simulink subsystem "F550_Dynamics_sub"  (R2024a)
settings: Solver=VariableStepAuto  StartTime=0.0  StopTime=10.0  RelTol=1e-3
undefined symbols (not defined in the file): armLength, Cd, Cmd, contact, control, ddx, ddy, ddz, dx, dy, dz, dzcg, g, Inertia, Inertia_inv, Mass, motorCr, motorJm, motorRpm0, motorTm, motorWb, p, pitch, q, r, roll, rotorCm, rotorCt, X, x0, Y, yaw, Z
libraries: matrix_library x2, shared6dof x1, simulink x1
settings Model: Creator=CNU_UASG  LastModifiedBy=CNU_UASG

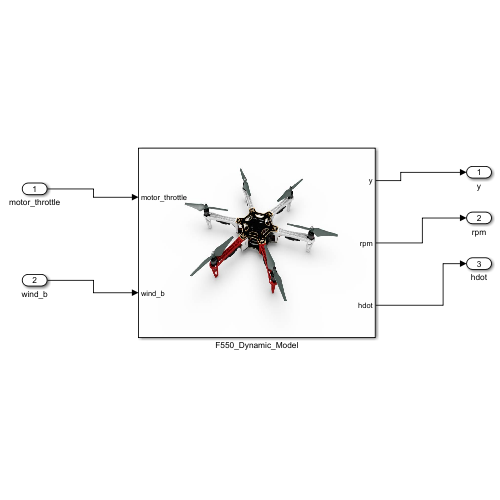
[thumbnail: Simulink's stored preview of the top-level diagram]
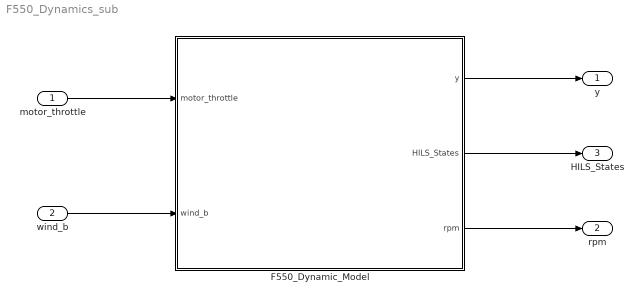
== system F550_Dynamics_sub ==
  motor_throttle : Inport
  wind_b : Inport  Port=2  PortDimensions=[3 1]
  F550_Dynamic_Model : Subsystem
      mask Display: image('F550.jpg');
  y : Outport
  rpm : Outport  Port=2
  HILS_States : Outport  Port=3
  wires:
  F550_Dynamic_Model/1(y) -> y/1
  F550_Dynamic_Model/3(rpm) -> rpm/1
  motor_throttle/1 -> F550_Dynamic_Model/1(motor_throttle)
  wind_b/1 -> F550_Dynamic_Model/2(wind_b)
  F550_Dynamic_Model/2(HILS_States) -> HILS_States/1

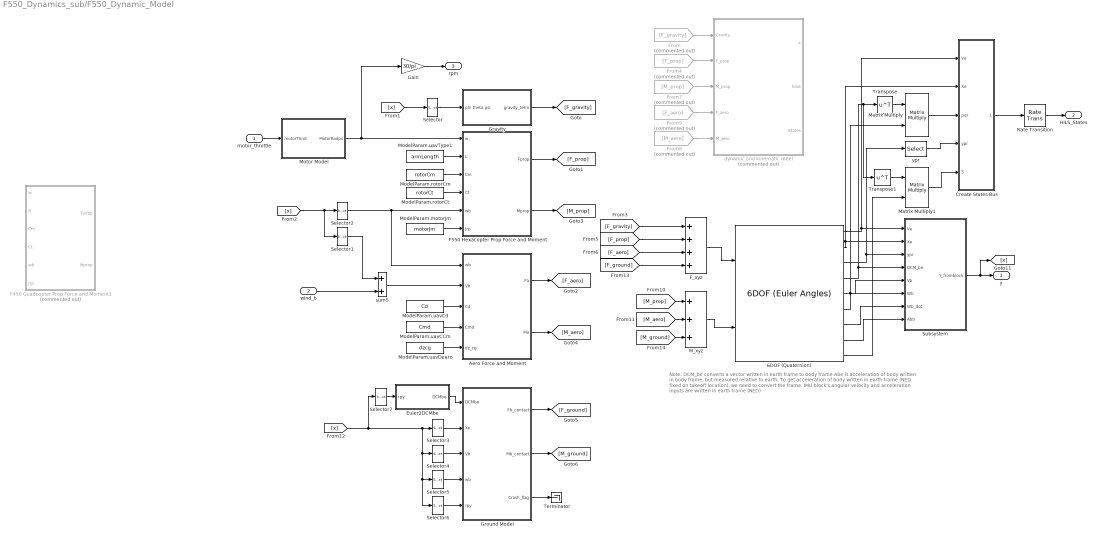
== system F550_Dynamics_sub/F550_Dynamic_Model ==
  note: Note:
      | DCM_be converts a vector written in earth frame to body frame
      | Abe is acceleration of body written in body frame, but measured relative to earth.
      | To get acceleration of body written in earth frame (NED fixed on takeoff location), we need to convert the frame.
      | IMU block's angular velocity and acceleration inputs are written in earth frame (NED)
  motor_throttle : Inport
  wind_b : Inport  Port=2
  6DOF (Quaternion) : shared6dof/6DOF (Euler Angles)  units=Metric (MKS)  mtype=Fixed  rep=Quaternion  xme_0=x0(10:12)  Vm_0=x0(1:3)  eul_0=x0(7:9)  pm_0=x0(4:6)  mass_0=Mass  mass_e=0.5  mass_f=2.0  inertia=Inertia  inertia_e=eye(3)  inertia_f=2*eye(3)  k_quat=1.0  vre_flag=on  abi_flag=on  aMode=0  xme_statename=''  Vm_statename=''  eul_statename=''  quat_statename=''  pm_statename=''  mass_statename=''
      settings: LibrarySourceBlock=aerolib6dof2/6DOF (Quaternion)
  Aero Force and Moment : MATLAB Function  TreatAsAtomicUnit=on
  Create States Bus : Subsystem
  Euler2DCMbe : MATLAB Function  TreatAsAtomicUnit=on
  F450 Quadcopter Prop Force and Moment1 : MATLAB Function  Commented=on  TreatAsAtomicUnit=on
  F550 Hexacopter Prop Force and Moment : MATLAB Function  TreatAsAtomicUnit=on
  F_xyz : Sum  Inputs=++++
  From : From  Commented=on  GotoTag=F_gravity
  From4 : From  Commented=on  GotoTag=F_prop
  From7 : From  Commented=on  GotoTag=M_prop
  From8 : From  Commented=on  GotoTag=M_aero
  From9 : From  Commented=on  GotoTag=F_aero
  Gain : Gain  Gain=30/pi
  Gravity : Subsystem
  Ground Model : Subsystem
  M_xyz : Sum  Inputs=+++
  Matrix Multiply : Product  Multiplication=Matrix(*)
  Matrix Multiply1 : Product  Multiplication=Matrix(*)
  ModelParam.motorJm : Constant  Value=motorJm
  ModelParam.rotorCm : Constant  Value=rotorCm
  ModelParam.rotorCt : Constant  Value=rotorCt
  ModelParam.uavCCm : Constant  Value=Cmd
  ModelParam.uavCd : Constant  Value=Cd
  ModelParam.uavDearo : Constant  Value=dzcg
  ModelParam.uavType1 : Constant  Value=armLength
  Motor Model : Subsystem
  Rate Transition : RateTransition  OutPortSampleTime=SampleTime
  Selector : Selector  InputPortWidth=12  IndexOptions=Index vector (dialog)  Indices=[7 8 9]  OutputSizes=1
  Selector1 : Selector  InputPortWidth=12  IndexOptions=Index vector (dialog)  Indices=[1 2 3]  OutputSizes=1
  Selector2 : Selector  InputPortWidth=12  IndexOptions=Index vector (dialog)  Indices=[4 5 6]  OutputSizes=1
  Selector3 : Selector  InputPortWidth=12  IndexOptions=Index vector (dialog)  Indices=[10 11 12]  OutputSizes=1
  Selector4 : Selector  InputPortWidth=12  IndexOptions=Index vector (dialog)  Indices=[1 2 3]  OutputSizes=1
  Selector5 : Selector  InputPortWidth=12  IndexOptions=Index vector (dialog)  Indices=[4 5 6]  OutputSizes=1
  Selector6 : Selector  InputPortWidth=12  IndexOptions=Index vector (dialog)  Indices=[7 8 9]  OutputSizes=1
  Selector7 : Selector  InputPortWidth=12  IndexOptions=Index vector (dialog)  Indices=[7 8 9]  OutputSizes=1
  Subsystem : Subsystem
  Terminator : Terminator
  Transpose : Math  Operator=transpose
  Transpose1 : Math  Operator=transpose
  dynamic and kinematic mdel : Subsystem  Commented=on
  sum5 : Sum  InputSameDT=on  SaturateOnIntegerOverflow=on  OutDataTypeStr=Inherit: Same as first input
  ypr : Selector  InputPortWidth=3  IndexOptions=Index vector (dialog)  Indices=[3 2 1]  OutputSizes=1
  y : Outport
  HILS_States : Outport  Port=2
  rpm : Outport  Port=3
  wires:
  Rate Transition/1 -> HILS_States/1
  [M_ground] -> M_xyz/3
  [F_ground] -> F_xyz/4
  Ground Model/3(Crash_flag) -> Terminator/1
  Ground Model/2(Mb_contact) -> [M_ground]
  Ground Model/1(Fb_contact) -> [F_ground]
  Selector7/1 -> Euler2DCMbe/1(rpy)
  Euler2DCMbe/1(DCMbe) -> Ground Model/1(DCMbe)
  Selector6/1 -> Ground Model/5(rpy)
  Selector5/1 -> Ground Model/4(wb)
  Selector4/1 -> Ground Model/3(Vb)
  Selector3/1 -> Ground Model/2(Xe)
  [x] -> Selector3/1, Selector4/1, Selector5/1, Selector6/1, Selector7/1
  6DOF (Quaternion)/9 -> Matrix Multiply1/2
  Transpose1/1 -> Matrix Multiply1/1
  Matrix Multiply1/1 -> Create States Bus/5(acc_lnav)
  ypr/1 -> Create States Bus/4(ypr)
  Transpose/1 -> Matrix Multiply/1
  Matrix Multiply/1 -> Create States Bus/3(pqr)
  Create States Bus/1(States) -> Rate Transition/1
  F_xyz/1 -> 6DOF (Quaternion)/1
  M_xyz/1 -> 6DOF (Quaternion)/2
  ModelParam.uavDearo/1 -> Aero Force and Moment/5(dz_cg)
  ModelParam.uavCCm/1 -> Aero Force and Moment/4(Cmd)
  ModelParam.uavCd/1 -> Aero Force and Moment/3(Cd)
  ModelParam.motorJm/1 -> F550 Hexacopter Prop Force and Moment/6(Jrp)
  ModelParam.uavType1/1 -> F550 Hexacopter Prop Force and Moment/2(L)
  ModelParam.rotorCt/1 -> F550 Hexacopter Prop Force and Moment/4(Ct)
  ModelParam.rotorCm/1 -> F550 Hexacopter Prop Force and Moment/3(Cm)
  motor_throttle/1 -> Motor Model/1(motorThrot)
  Gain/1 -> rpm/1
  [x] -> Selector/1
  [x] -> Selector2/1, Selector1/1
  Motor Model/1(MotorRadps) -> F550 Hexacopter Prop Force and Moment/1(w), Gain/1
  wind_b/1 -> sum5/2
  sum5/1 -> Aero Force and Moment/2(Vb)
  Selector/1 -> Gravity/1(phi theta psi)
  Selector2/1 -> Aero Force and Moment/1(wb), F550 Hexacopter Prop Force and Moment/5(wb)
  Selector1/1 -> sum5/1
  6DOF (Quaternion)/1 -> Subsystem/1(Ve), Create States Bus/1(Ve)
  6DOF (Quaternion)/2 -> Subsystem/2(Xe), Create States Bus/2(Xe)
  6DOF (Quaternion)/3 -> ypr/1, Subsystem/3(ypr)
  6DOF (Quaternion)/4 -> Transpose1/1, Transpose/1, Subsystem/4(DCM_be)
  6DOF (Quaternion)/5 -> Subsystem/5(Vb)
  6DOF (Quaternion)/6 -> Matrix Multiply/2, Subsystem/6(Wb)
  6DOF (Quaternion)/7 -> Subsystem/7(Wb_dot)
  6DOF (Quaternion)/8 -> Subsystem/8(Abb)
  Gravity/1(gravity_term) -> [F_gravity]
  From/1 -> dynamic and kinematic mdel/1(Gravity)
  F550 Hexacopter Prop Force and Moment/1(Fprop) -> [F_prop]
  From4/1 -> dynamic and kinematic mdel/2(F_prop)
  Aero Force and Moment/1(Fa) -> [F_aero]
  F550 Hexacopter Prop Force and Moment/2(Mprop) -> [M_prop]
  Aero Force and Moment/2(Ma) -> [M_aero]
  [F_prop] -> F_xyz/2
  [F_gravity] -> F_xyz/1
  [F_aero] -> F_xyz/3
  From7/1 -> dynamic and kinematic mdel/3(M_prop)
  From8/1 -> dynamic and kinematic mdel/5(M_aero)
  From9/1 -> dynamic and kinematic mdel/4(F_aero)
  [M_prop] -> M_xyz/1
  [M_aero] -> M_xyz/2
  Subsystem/1(Y_fromblock) -> y/1, [x]

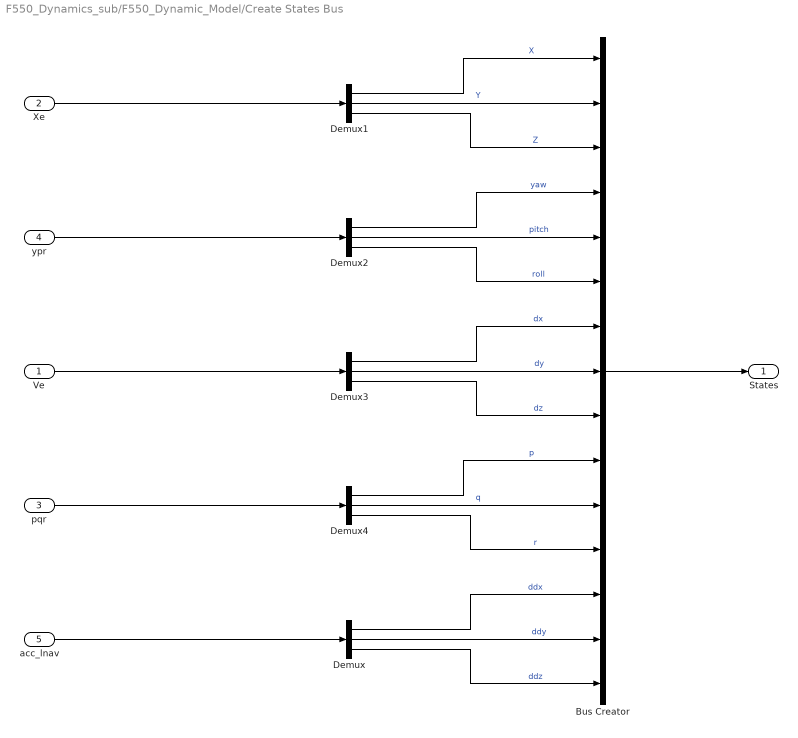
== system F550_Dynamics_sub/F550_Dynamic_Model/Create States Bus ==
  Ve : Inport
  Xe : Inport  Port=2
  pqr : Inport  Port=3
  ypr : Inport  Port=4
  acc_lnav : Inport  Port=5
  Bus Creator : BusCreator  Inputs=X,Y,Z,yaw,pitch,roll,dx,dy,dz,p,q,r,ddx,ddy,ddz
  Demux{,1..4} (5 alike) : Demux  Outputs=3
  States : Outport
  wires:
  acc_lnav/1 -> Demux/1
  pqr/1 -> Demux4/1
  Ve/1 -> Demux3/1
  ypr/1 -> Demux2/1
  Xe/1 -> Demux1/1
  Demux/1 -> Bus Creator/13  "ddx"
  Demux/2 -> Bus Creator/14  "ddy"
  Demux/3 -> Bus Creator/15  "ddz"
  Bus Creator/1 -> States/1
  Demux4/1 -> Bus Creator/10  "p"
  Demux4/3 -> Bus Creator/12  "r"
  Demux3/3 -> Bus Creator/9  "dz"
  Demux4/2 -> Bus Creator/11  "q"
  Demux3/1 -> Bus Creator/7  "dx"
  Demux1/3 -> Bus Creator/3  "Z"
  Demux2/1 -> Bus Creator/4  "yaw"
  Demux2/3 -> Bus Creator/6  "roll"
  Demux3/2 -> Bus Creator/8  "dy"
  Demux2/2 -> Bus Creator/5  "pitch"
  Demux1/2 -> Bus Creator/2  "Y"
  Demux1/1 -> Bus Creator/1  "X"

== system F550_Dynamics_sub/F550_Dynamic_Model/Gravity ==
  note: Gravaity
  phi theta psi : Inport
  . : Gain  Gain=g*Mass  SaturateOnIntegerOverflow=on  OutDataTypeStr=Inherit: Same as input  ParamDataTypeStr=Inherit: Same as input
  Mux : Mux  Inputs=3
  psidot2 : Fcn  Expr=cos(u[2])*cos(u[1])
  t : Fcn  Expr=-sin(u[2])
  tetadot : Fcn  Expr=cos(u[2])*sin(u[1])
  gravity_term : Outport  InitialOutput=0  VectorParamsAs1DForOutWhenUnconnected=off
  wires:
  t/1 -> Mux/1
  psidot2/1 -> Mux/3
  tetadot/1 -> Mux/2
  Mux/1 -> ./1
  phi theta psi/1 -> tetadot/1, t/1, psidot2/1
  ./1 -> gravity_term/1

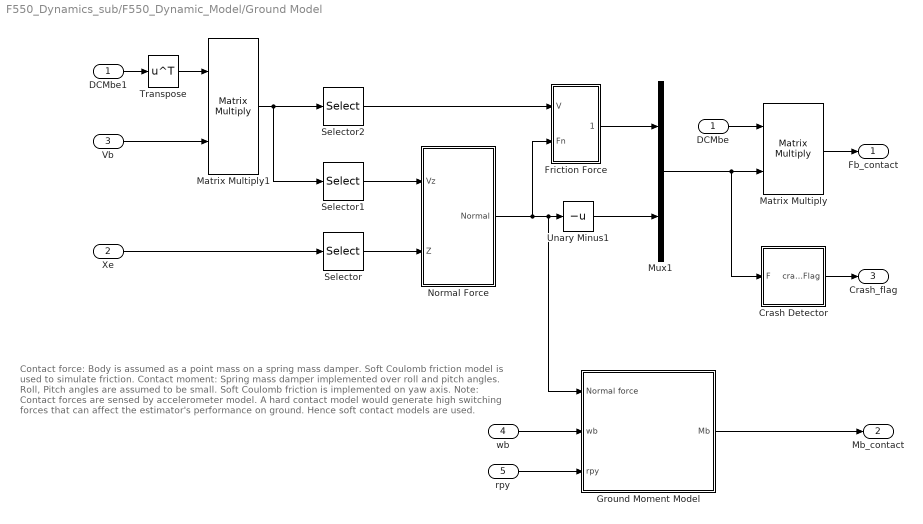
== system F550_Dynamics_sub/F550_Dynamic_Model/Ground Model ==
  note: Contact force:
      | Body is assumed as a point mass on a spring mass damper. Soft Coulomb friction model is used to simulate friction.
      |
      | Contact moment:
      | Spring mass damper implemented over roll and pitch angles. Roll, Pitch angles are assumed to be small.
      | Soft Coulomb friction is implemented on yaw axis.
      |
      | Note:
      | Contact forces are sensed by accelerometer model. A hard contact model would generate high switching forces that can affect the estimator's performance on ground. Hence soft contact models are used.
  DCMbe : Inport
  Xe : Inport  Port=2
  Vb : Inport  Port=3
  wb : Inport  Port=4
  rpy : Inport  Port=5
  Crash Detector : Subsystem
  DCMbe1 : InportShadow
  Friction Force : Subsystem
  Ground Moment Model : Subsystem
  Matrix Multiply : Product  Multiplication=Matrix(*)
  Matrix Multiply1 : Product  Multiplication=Matrix(*)
  Mux1 : Mux  Inputs=2
  Normal Force : Subsystem
  Selector : Selector  InputPortWidth=3  IndexOptions=Index vector (dialog)  Indices=[3]  OutputSizes=1
  Selector1 : Selector  InputPortWidth=3  IndexOptions=Index vector (dialog)  Indices=[3]  OutputSizes=1
  Selector2 : Selector  InputPortWidth=3  IndexOptions=Index vector (dialog)  Indices=[1,2]  OutputSizes=1
  Transpose : Math  Operator=transpose
  Unary Minus1 : UnaryMinus
  Fb_contact : Outport
  Mb_contact : Outport  Port=2
  Crash_flag : Outport  Port=3
  wires:
  Ground Moment Model/1(Mb) -> Mb_contact/1
  rpy/1 -> Ground Moment Model/3(rpy)
  wb/1 -> Ground Moment Model/2(wb)
  Matrix Multiply1/1 -> Selector2/1, Selector1/1
  Vb/1 -> Matrix Multiply1/2
  Transpose/1 -> Matrix Multiply1/1
  DCMbe1/1 -> Transpose/1
  Friction Force/1(Friction) -> Mux1/1
  Selector2/1 -> Friction Force/1(V)
  Unary Minus1/1 -> Mux1/2
  Mux1/1 -> Matrix Multiply/2, Crash Detector/1(F)
  Normal Force/1(Normal) -> Friction Force/2(Fn), Unary Minus1/1, Ground Moment Model/1(Normal force)
  Matrix Multiply/1 -> Fb_contact/1
  DCMbe/1 -> Matrix Multiply/1
  Selector/1 -> Normal Force/2(Z)
  Selector1/1 -> Normal Force/1(Vz)
  Xe/1 -> Selector/1
  Crash Detector/1(crashFlag) -> Crash_flag/1

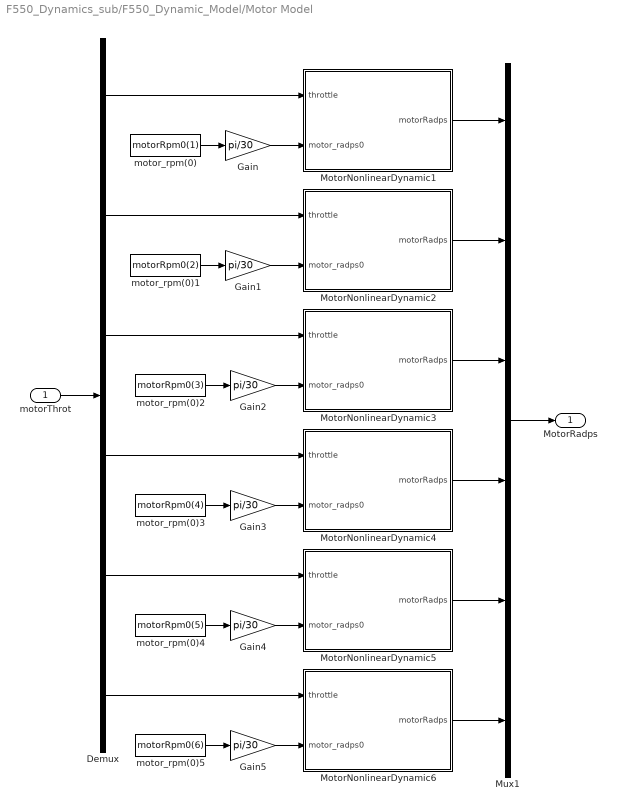
== system F550_Dynamics_sub/F550_Dynamic_Model/Motor Model ==
  motorThrot : Inport
  Demux : Demux  Outputs=6
  Gain{,1..5} (6 alike) : Gain  Gain=pi/30
  MotorNonlinearDynamic1 : Subsystem  TreatAsAtomicUnit=on
  MotorNonlinearDynamic2 : Subsystem  TreatAsAtomicUnit=on
  MotorNonlinearDynamic3 : Subsystem  TreatAsAtomicUnit=on
  MotorNonlinearDynamic4 : Subsystem  TreatAsAtomicUnit=on
  MotorNonlinearDynamic5 : Subsystem  TreatAsAtomicUnit=on
  MotorNonlinearDynamic6 : Subsystem  TreatAsAtomicUnit=on
  Mux1 : Mux  Inputs=6
  motor_rpm(0) : Constant  Value=motorRpm0(1)
  motor_rpm(0)1 : Constant  Value=motorRpm0(2)
  motor_rpm(0)2 : Constant  Value=motorRpm0(3)
  motor_rpm(0)3 : Constant  Value=motorRpm0(4)
  motor_rpm(0)4 : Constant  Value=motorRpm0(5)
  motor_rpm(0)5 : Constant  Value=motorRpm0(6)
  MotorRadps : Outport  VectorParamsAs1DForOutWhenUnconnected=off
  wires:
  motorThrot/1 -> Demux/1
  Demux/4 -> MotorNonlinearDynamic4/1(throttle)
  motor_rpm(0)/1 -> Gain/1
  MotorNonlinearDynamic3/1(motorRadps) -> Mux1/3
  MotorNonlinearDynamic2/1(motorRadps) -> Mux1/2
  Mux1/1 -> MotorRadps/1
  Demux/2 -> MotorNonlinearDynamic2/1(throttle)
  Demux/3 -> MotorNonlinearDynamic3/1(throttle)
  Demux/1 -> MotorNonlinearDynamic1/1(throttle)
  MotorNonlinearDynamic4/1(motorRadps) -> Mux1/4
  MotorNonlinearDynamic1/1(motorRadps) -> Mux1/1
  Gain/1 -> MotorNonlinearDynamic1/2(motor_radps0)
  motor_rpm(0)1/1 -> Gain1/1
  Gain1/1 -> MotorNonlinearDynamic2/2(motor_radps0)
  motor_rpm(0)2/1 -> Gain2/1
  Gain2/1 -> MotorNonlinearDynamic3/2(motor_radps0)
  motor_rpm(0)3/1 -> Gain3/1
  Gain3/1 -> MotorNonlinearDynamic4/2(motor_radps0)
  Gain4/1 -> MotorNonlinearDynamic5/2(motor_radps0)
  motor_rpm(0)4/1 -> Gain4/1
  Demux/5 -> MotorNonlinearDynamic5/1(throttle)
  Gain5/1 -> MotorNonlinearDynamic6/2(motor_radps0)
  motor_rpm(0)5/1 -> Gain5/1
  Demux/6 -> MotorNonlinearDynamic6/1(throttle)
  MotorNonlinearDynamic5/1(motorRadps) -> Mux1/5
  MotorNonlinearDynamic6/1(motorRadps) -> Mux1/6

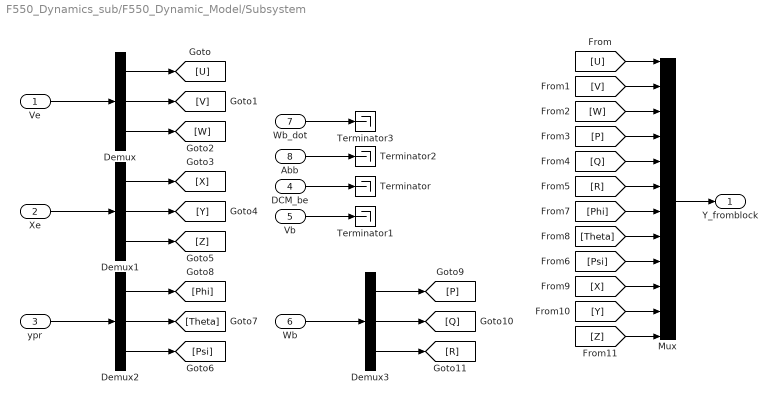
== system F550_Dynamics_sub/F550_Dynamic_Model/Subsystem ==
  Ve : Inport
  Xe : Inport  Port=2
  ypr : Inport  Port=3
  DCM_be : Inport  Port=4
  Vb : Inport  Port=5
  Wb : Inport  Port=6
  Wb_dot : Inport  Port=7
  Abb : Inport  Port=8
  Demux{,1..3} (4 alike) : Demux  Outputs=3
  Mux : Mux  Inputs=12
  Terminator{,1..3} (4 alike) : Terminator
  Y_fromblock : Outport
  wires:
  Demux2/3 -> [Psi]
  Demux2/1 -> [Phi]
  Ve/1 -> Demux/1
  Demux/1 -> [U]
  Demux/3 -> [W]
  Demux/2 -> [V]
  Xe/1 -> Demux1/1
  Demux1/1 -> [X]
  Demux1/2 -> [Y]
  Demux1/3 -> [Z]
  ypr/1 -> Demux2/1
  Demux2/2 -> [Theta]
  DCM_be/1 -> Terminator/1
  Demux3/1 -> [P]
  Demux3/2 -> [Q]
  Demux3/3 -> [R]
  Wb/1 -> Demux3/1
  Vb/1 -> Terminator1/1
  Abb/1 -> Terminator2/1
  Wb_dot/1 -> Terminator3/1
  Mux/1 -> Y_fromblock/1
  [U] -> Mux/1
  [V] -> Mux/2
  [W] -> Mux/3
  [P] -> Mux/4
  [Q] -> Mux/5
  [R] -> Mux/6
  [Phi] -> Mux/7
  [Theta] -> Mux/8
  [Psi] -> Mux/9
  [X] -> Mux/10
  [Y] -> Mux/11
  [Z] -> Mux/12

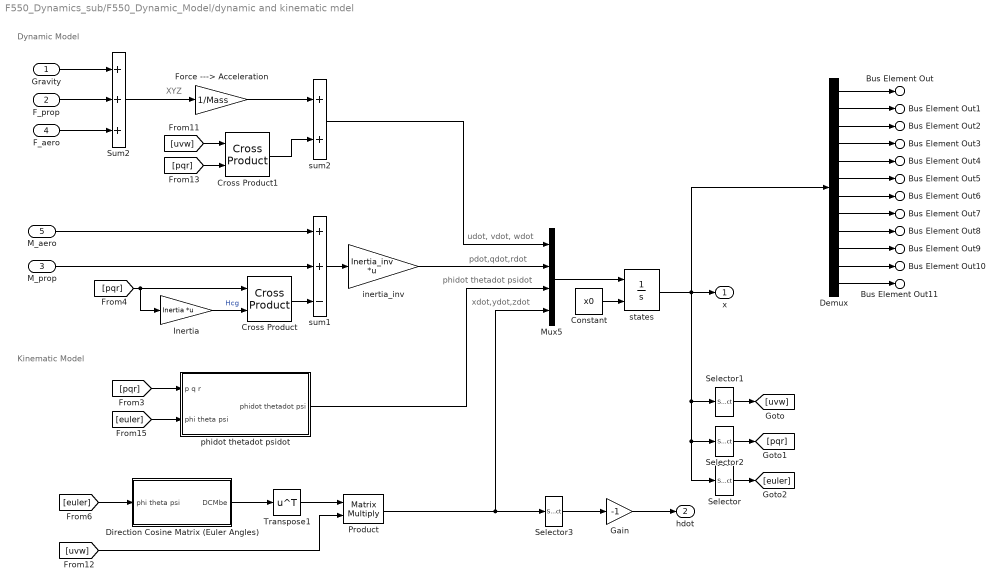
== system F550_Dynamics_sub/F550_Dynamic_Model/dynamic and kinematic mdel ==
  note: Kinematic Model
  note: udot, vdot, wdot
  note: pdot,qdot,rdot
  note: phidot thetadot psidot
  note: xdot,ydot,zdot
  note: XYZ
  note: Dynamic Model
  Gravity : Inport
  F_prop : Inport  Port=2
  M_prop : Inport  Port=3
  F_aero : Inport  Port=4
  M_aero : Inport  Port=5
  Constant : Constant  Value=x0
  Cross Product : matrix_library/Cross Product
  Cross Product1 : matrix_library/Cross Product
  Demux : Demux  Outputs=12
  Direction Cosine Matrix (Euler Angles) : Subsystem
  Force ---> Acceleration : Gain  Gain=1/Mass  SaturateOnIntegerOverflow=on  OutDataTypeStr=Inherit: Same as input  ParamDataTypeStr=Inherit: Same as input
  Gain : Gain  Gain=-1
  Inertia : Gain  Gain=Inertia  Multiplication=Matrix(K*u)
  Mux5 : Mux
  Product : Product  Multiplication=Matrix(*)  InputSameDT=on  RndMeth=Zero  SaturateOnIntegerOverflow=on  OutDataTypeStr=Inherit: Same as first input
  Selector : Selector  InputPortWidth=12  IndexOptions=Index vector (dialog)  Indices=[7 8 9]  OutputSizes=1
  Selector1 : Selector  InputPortWidth=12  IndexOptions=Index vector (dialog)  Indices=[1 2 3]  OutputSizes=1
  Selector2 : Selector  InputPortWidth=12  IndexOptions=Index vector (dialog)  Indices=[4 5 6]  OutputSizes=1
  Selector3 : Selector  InputPortWidth=3  IndexOptions=Index vector (dialog)  Indices=3  OutputSizes=1
  Sum2 : Sum  Inputs=+++  InputSameDT=on  SaturateOnIntegerOverflow=on  OutDataTypeStr=Inherit: Same as first input
  Transpose1 : Math  Operator=transpose  SignedPower=on
  inertia_inv : Gain  Gain=Inertia_inv  Multiplication=Matrix(K*u)
  phidot thetadot psidot : Subsystem
  states : Integrator  InitialConditionSource=external  InitialCondition=x0
  sum1 : Sum  Inputs=++-  InputSameDT=on  SaturateOnIntegerOverflow=on  OutDataTypeStr=Inherit: Same as first input
  sum2 : Sum  InputSameDT=on  SaturateOnIntegerOverflow=on  OutDataTypeStr=Inherit: Same as first input
  x : Outport  VectorParamsAs1DForOutWhenUnconnected=off
  hdot : Outport  Port=2  VectorParamsAs1DForOutWhenUnconnected=off
  Bus Element Out : Outport  Port=3  PortName=States  Element=U
  Bus Element Out1 : Outport  Port=3  PortName=States  Element=V
  Bus Element Out2 : Outport  Port=3  PortName=States  Element=W
  Bus Element Out3 : Outport  Port=3  PortName=States  Element=P
  Bus Element Out4 : Outport  Port=3  PortName=States  Element=Q
  Bus Element Out5 : Outport  Port=3  PortName=States  Element=R
  Bus Element Out6 : Outport  Port=3  PortName=States  Element=Phi
  Bus Element Out7 : Outport  Port=3  PortName=States  Element=Theta
  Bus Element Out8 : Outport  Port=3  PortName=States  Element=Psi
  Bus Element Out9 : Outport  Port=3  PortName=States  Element=X
  Bus Element Out10 : Outport  Port=3  PortName=States  Element=Y
  Bus Element Out11 : Outport  Port=3  PortName=States  Element=Z
  wires:
  [euler] -> Direction Cosine Matrix (Euler Angles)/1(phi theta psi)
  [uvw] -> Product/2
  Direction Cosine Matrix (Euler Angles)/1(DCMbe) -> Transpose1/1
  Transpose1/1 -> Product/1
  Gravity/1 -> Sum2/1
  M_prop/1 -> sum1/2
  Cross Product/1 -> sum1/3
  M_aero/1 -> sum1/1
  F_aero/1 -> Sum2/3
  F_prop/1 -> Sum2/2
  Sum2/1 -> Force ---> Acceleration/1
  Force ---> Acceleration/1 -> sum2/1
  Cross Product1/1 -> sum2/2
  sum1/1 -> inertia_inv/1
  Inertia/1 -> Cross Product/2  "Hcg"
  phidot thetadot psidot/1(phidot thetadot psi) -> Mux5/3
  sum2/1 -> Mux5/1
  inertia_inv/1 -> Mux5/2
  Mux5/1 -> states/1
  [pqr] -> Inertia/1, Cross Product/1
  [uvw] -> Cross Product1/1
  [pqr] -> Cross Product1/2
  [euler] -> phidot thetadot psidot/2(phi theta psi)
  Product/1 -> Selector3/1, Mux5/4
  [pqr] -> phidot thetadot psidot/1(p q r)
  Selector2/1 -> [pqr]
  states/1 -> Demux/1, Selector1/1, Selector/1, Selector2/1, x/1
  Selector1/1 -> [uvw]
  Constant/1 -> states/2
  Selector/1 -> [euler]
  Selector3/1 -> Gain/1
  Gain/1 -> hdot/1
  Demux/1 -> Bus Element Out/1
  Demux/2 -> Bus Element Out1/1
  Demux/3 -> Bus Element Out2/1
  Demux/5 -> Bus Element Out4/1
  Demux/4 -> Bus Element Out3/1
  Demux/6 -> Bus Element Out5/1
  Demux/7 -> Bus Element Out6/1
  Demux/8 -> Bus Element Out7/1
  Demux/9 -> Bus Element Out8/1
  Demux/10 -> Bus Element Out9/1
  Demux/11 -> Bus Element Out10/1
  Demux/12 -> Bus Element Out11/1

== system F550_Dynamics_sub/F550_Dynamic_Model/Ground Model/Crash Detector ==
  F : Inport
  Compare To Constant : simulink/Logic and Bit Operations/Compare To Constant  relop=>  const=100  OutDataTypeStr=boolean
  Gain : Gain  Gain=1/Mass/g
  norm1 : Subsystem
  crashFlag : Outport
  wires:
  Gain/1 -> Compare To Constant/1  "g's"
  Compare To Constant/1 -> crashFlag/1
  norm1/1(Out1) -> Gain/1
  F/1 -> norm1/1(F)

== system F550_Dynamics_sub/F550_Dynamic_Model/Ground Model/Friction Force ==
  V : Inport
  Fn : Inport  Port=2
  Product : Product
  Saturation : Saturate  UpperLimit=contact.translation.maxFriction  LowerLimit=-contact.translation.maxFriction
  Soft Coulomb Friction : Subsystem
  Unary Minus : UnaryMinus
  Friction : Outport
  wires:
  Saturation/1 -> Friction/1
  Unary Minus/1 -> Saturation/1
  V/1 -> Soft Coulomb Friction/1(In1)
  Product/1 -> Unary Minus/1
  Soft Coulomb Friction/1(Out1) -> Product/1
  Fn/1 -> Product/2

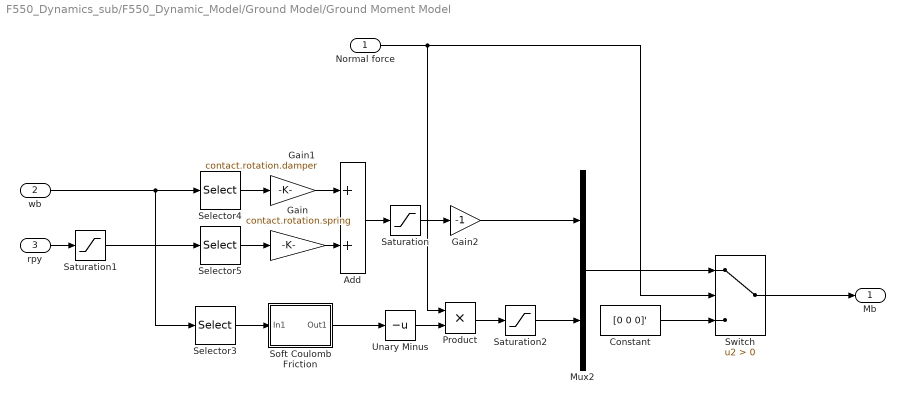
== system F550_Dynamics_sub/F550_Dynamic_Model/Ground Model/Ground Moment Model ==
  Normal force : Inport
  wb : Inport  Port=2
  rpy : Inport  Port=3
  Add : Sum
  Constant : Constant  Value=[0 0 0]'
  Gain : Gain  Gain=contact.rotation.spring
  Gain1 : Gain  Gain=contact.rotation.damper
  Gain2 : Gain  Gain=-1
  Mux2 : Mux  Inputs=2
  Product : Product
  Saturation : Saturate  UpperLimit=control.rotation.maxMoment  LowerLimit=-control.rotation.maxMoment
  Saturation1 : Saturate  UpperLimit=20*pi/180  LowerLimit=-20*pi/180
  Saturation2 : Saturate  UpperLimit=control.rotation.maxMoment  LowerLimit=-control.rotation.maxMoment
  Selector3 : Selector  InputPortWidth=3  IndexOptions=Index vector (dialog)  Indices=[3]  OutputSizes=1
  Selector4 : Selector  InputPortWidth=3  IndexOptions=Index vector (dialog)  Indices=[1, 2]  OutputSizes=1
  Selector5 : Selector  InputPortWidth=3  IndexOptions=Index vector (dialog)  Indices=[1, 2]  OutputSizes=1
  Soft Coulomb Friction : Subsystem
  Switch : Switch  Criteria=u2 > Threshold  SaturateOnIntegerOverflow=off  InputSameDT=off
  Unary Minus : UnaryMinus
  Mb : Outport
  wires:
  Saturation2/1 -> Mux2/2
  Product/1 -> Saturation2/1
  Unary Minus/1 -> Product/2
  Soft Coulomb Friction/1(Out1) -> Unary Minus/1
  Selector3/1 -> Soft Coulomb Friction/1(In1)
  wb/1 -> Selector3/1, Selector4/1
  Saturation1/1 -> Selector5/1
  rpy/1 -> Saturation1/1
  Normal force/1 -> Switch/2, Product/1
  Mux2/1 -> Switch/1
  Switch/1 -> Mb/1
  Selector5/1 -> Gain/1
  Constant/1 -> Switch/3
  Gain1/1 -> Add/1
  Selector4/1 -> Gain1/1
  Saturation/1 -> Gain2/1
  Gain/1 -> Add/2
  Add/1 -> Saturation/1
  Gain2/1 -> Mux2/1

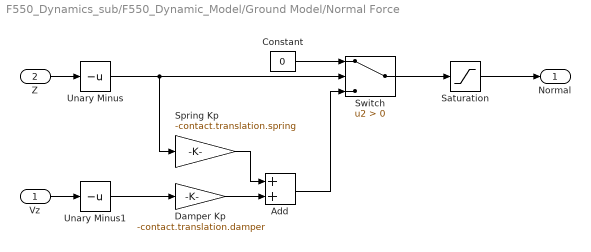
== system F550_Dynamics_sub/F550_Dynamic_Model/Ground Model/Normal Force ==
  Vz : Inport
  Z : Inport  Port=2
  Add : Sum
  Constant : Constant  Value=0
  Damper Kp : Gain  Gain=-contact.translation.damper
  Saturation : Saturate  UpperLimit=contact.translation.maxNormal  LowerLimit=0
  Spring Kp : Gain  Gain=-contact.translation.spring
  Switch : Switch  Criteria=u2 > Threshold  SaturateOnIntegerOverflow=off  InputSameDT=off
  Unary Minus : UnaryMinus
  Unary Minus1 : UnaryMinus
  Normal : Outport
  wires:
  Unary Minus1/1 -> Damper Kp/1
  Unary Minus/1 -> Switch/2, Spring Kp/1
  Saturation/1 -> Normal/1
  Vz/1 -> Unary Minus1/1
  Spring Kp/1 -> Add/1
  Add/1 -> Switch/3
  Damper Kp/1 -> Add/2
  Switch/1 -> Saturation/1
  Z/1 -> Unary Minus/1
  Constant/1 -> Switch/1

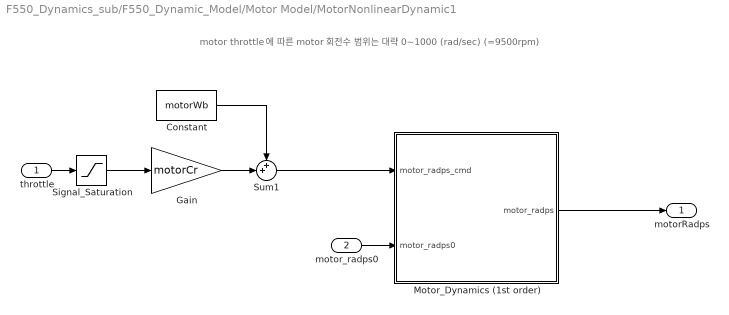
== system F550_Dynamics_sub/F550_Dynamic_Model/Motor Model/MotorNonlinearDynamic1 ==
  note: motor throttle 에 따른 motor 회전수 범위는 대략 0~1000 (rad/sec) (=9500rpm)
  throttle : Inport
  motor_radps0 : Inport  Port=2
  Constant : Constant  Value=motorWb
  Gain : Gain  Gain=motorCr
  Motor_Dynamics (1st order) : Subsystem  TreatAsAtomicUnit=on
  Signal_Saturation : Saturate  UpperLimit=0.95  LowerLimit=0
      settings: AttributesFormatString=%<LowerLimit>~%<UpperLimit>
  Sum1 : Sum  Inputs=++|
  motorRadps : Outport  VectorParamsAs1DForOutWhenUnconnected=off
  wires:
  Motor_Dynamics (1st order)/1(motor_radps) -> motorRadps/1
  motor_radps0/1 -> Motor_Dynamics (1st order)/2(motor_radps0)
  Constant/1 -> Sum1/1
  Gain/1 -> Sum1/2
  Signal_Saturation/1 -> Gain/1
  Sum1/1 -> Motor_Dynamics (1st order)/1(motor_radps_cmd)
  throttle/1 -> Signal_Saturation/1

== system F550_Dynamics_sub/F550_Dynamic_Model/Motor Model/MotorNonlinearDynamic2 ==
  note: motor throttle 에 따른 motor 회전수 범위는 대략 0~1000 (rad/sec) (=9500rpm)
  throttle : Inport
  motor_radps0 : Inport  Port=2
  Constant : Constant  Value=motorWb
  Gain : Gain  Gain=motorCr
  Motor_Dynamics (1st order) : Subsystem  TreatAsAtomicUnit=on
  Signal_Saturation : Saturate  UpperLimit=0.95  LowerLimit=0
      settings: AttributesFormatString=%<LowerLimit>~%<UpperLimit>
  Sum1 : Sum  Inputs=++|
  motorRadps : Outport  VectorParamsAs1DForOutWhenUnconnected=off
  wires:
  throttle/1 -> Signal_Saturation/1
  Sum1/1 -> Motor_Dynamics (1st order)/1(motor_radps_cmd)
  Signal_Saturation/1 -> Gain/1
  Gain/1 -> Sum1/2
  Constant/1 -> Sum1/1
  motor_radps0/1 -> Motor_Dynamics (1st order)/2(motor_radps0)
  Motor_Dynamics (1st order)/1(motor_radps) -> motorRadps/1

== system F550_Dynamics_sub/F550_Dynamic_Model/Motor Model/MotorNonlinearDynamic3 ==
  note: motor throttle 에 따른 motor 회전수 범위는 대략 0~1000 (rad/sec) (=9500rpm)
  throttle : Inport
  motor_radps0 : Inport  Port=2
  Constant : Constant  Value=motorWb
  Gain : Gain  Gain=motorCr
  Motor_Dynamics (1st order) : Subsystem  TreatAsAtomicUnit=on
  Signal_Saturation : Saturate  UpperLimit=0.95  LowerLimit=0
      settings: AttributesFormatString=%<LowerLimit>~%<UpperLimit>
  Sum1 : Sum  Inputs=++|
  motorRadps : Outport  VectorParamsAs1DForOutWhenUnconnected=off
  wires:
  Motor_Dynamics (1st order)/1(motor_radps) -> motorRadps/1
  motor_radps0/1 -> Motor_Dynamics (1st order)/2(motor_radps0)
  Constant/1 -> Sum1/1
  Gain/1 -> Sum1/2
  Signal_Saturation/1 -> Gain/1
  Sum1/1 -> Motor_Dynamics (1st order)/1(motor_radps_cmd)
  throttle/1 -> Signal_Saturation/1

== system F550_Dynamics_sub/F550_Dynamic_Model/Motor Model/MotorNonlinearDynamic4 ==
  note: motor throttle 에 따른 motor 회전수 범위는 대략 0~1000 (rad/sec) (=9500rpm)
  throttle : Inport
  motor_radps0 : Inport  Port=2
  Constant : Constant  Value=motorWb
  Gain : Gain  Gain=motorCr
  Motor_Dynamics (1st order) : Subsystem  TreatAsAtomicUnit=on
  Signal_Saturation : Saturate  UpperLimit=0.95  LowerLimit=0
      settings: AttributesFormatString=%<LowerLimit>~%<UpperLimit>
  Sum1 : Sum  Inputs=++|
  motorRadps : Outport  VectorParamsAs1DForOutWhenUnconnected=off
  wires:
  throttle/1 -> Signal_Saturation/1
  Sum1/1 -> Motor_Dynamics (1st order)/1(motor_radps_cmd)
  Signal_Saturation/1 -> Gain/1
  Gain/1 -> Sum1/2
  Constant/1 -> Sum1/1
  motor_radps0/1 -> Motor_Dynamics (1st order)/2(motor_radps0)
  Motor_Dynamics (1st order)/1(motor_radps) -> motorRadps/1

== system F550_Dynamics_sub/F550_Dynamic_Model/Motor Model/MotorNonlinearDynamic5 ==
  note: motor throttle 에 따른 motor 회전수 범위는 대략 0~1000 (rad/sec) (=9500rpm)
  throttle : Inport
  motor_radps0 : Inport  Port=2
  Constant : Constant  Value=motorWb
  Gain : Gain  Gain=motorCr
  Motor_Dynamics (1st order) : Subsystem  TreatAsAtomicUnit=on
  Signal_Saturation : Saturate  UpperLimit=0.95  LowerLimit=0
      settings: AttributesFormatString=%<LowerLimit>~%<UpperLimit>
  Sum1 : Sum  Inputs=++|
  motorRadps : Outport  VectorParamsAs1DForOutWhenUnconnected=off
  wires:
  throttle/1 -> Signal_Saturation/1
  Sum1/1 -> Motor_Dynamics (1st order)/1(motor_radps_cmd)
  Signal_Saturation/1 -> Gain/1
  Gain/1 -> Sum1/2
  Constant/1 -> Sum1/1
  motor_radps0/1 -> Motor_Dynamics (1st order)/2(motor_radps0)
  Motor_Dynamics (1st order)/1(motor_radps) -> motorRadps/1

== system F550_Dynamics_sub/F550_Dynamic_Model/Motor Model/MotorNonlinearDynamic6 ==
  note: motor throttle 에 따른 motor 회전수 범위는 대략 0~1000 (rad/sec) (=9500rpm)
  throttle : Inport
  motor_radps0 : Inport  Port=2
  Constant : Constant  Value=motorWb
  Gain : Gain  Gain=motorCr
  Motor_Dynamics (1st order) : Subsystem  TreatAsAtomicUnit=on
  Signal_Saturation : Saturate  UpperLimit=0.95  LowerLimit=0
      settings: AttributesFormatString=%<LowerLimit>~%<UpperLimit>
  Sum1 : Sum  Inputs=++|
  motorRadps : Outport  VectorParamsAs1DForOutWhenUnconnected=off
  wires:
  throttle/1 -> Signal_Saturation/1
  Sum1/1 -> Motor_Dynamics (1st order)/1(motor_radps_cmd)
  Signal_Saturation/1 -> Gain/1
  Gain/1 -> Sum1/2
  Constant/1 -> Sum1/1
  motor_radps0/1 -> Motor_Dynamics (1st order)/2(motor_radps0)
  Motor_Dynamics (1st order)/1(motor_radps) -> motorRadps/1

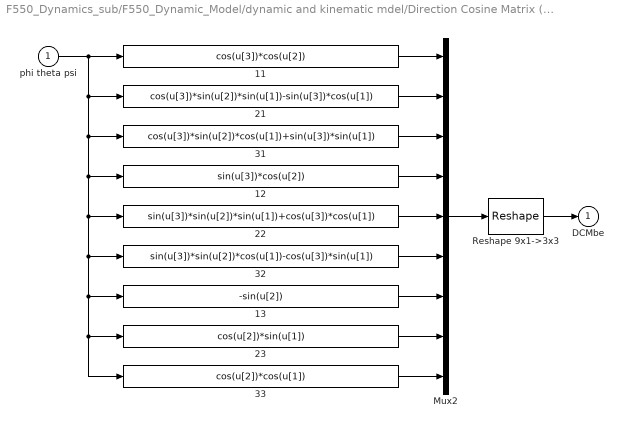
== system F550_Dynamics_sub/F550_Dynamic_Model/dynamic and kinematic mdel/Direction Cosine Matrix (Euler Angles) ==
  phi theta psi : Inport
  11 : Fcn  Expr=cos(u[3])*cos(u[2])
  12 : Fcn  Expr=sin(u[3])*cos(u[2])
  13 : Fcn  Expr=-sin(u[2])
  21 : Fcn  Expr=cos(u[3])*sin(u[2])*sin(u[1])-sin(u[3])*cos(u[1])
  22 : Fcn  Expr=sin(u[3])*sin(u[2])*sin(u[1])+cos(u[3])*cos(u[1])
  23 : Fcn  Expr=cos(u[2])*sin(u[1])
  31 : Fcn  Expr=cos(u[3])*sin(u[2])*cos(u[1])+sin(u[3])*sin(u[1])
  32 : Fcn  Expr=sin(u[3])*sin(u[2])*cos(u[1])-cos(u[3])*sin(u[1])
  33 : Fcn  Expr=cos(u[2])*cos(u[1])
  Mux2 : Mux  Inputs=9
  Reshape 9x1->3x3 : Reshape  OutputDimensionality=Customize  OutputDimensions=[3,3]
  DCMbe : Outport  InitialOutput=0  VectorParamsAs1DForOutWhenUnconnected=off
  wires:
  31/1 -> Mux2/3
  Mux2/1 -> Reshape 9x1->3x3/1
  11/1 -> Mux2/1
  12/1 -> Mux2/4
  13/1 -> Mux2/7
  21/1 -> Mux2/2
  Reshape 9x1->3x3/1 -> DCMbe/1
  23/1 -> Mux2/8
  33/1 -> Mux2/9
  22/1 -> Mux2/5
  32/1 -> Mux2/6
  phi theta psi/1 -> 23/1, 33/1, 13/1, 32/1, 22/1, 12/1, 31/1, 21/1, 11/1

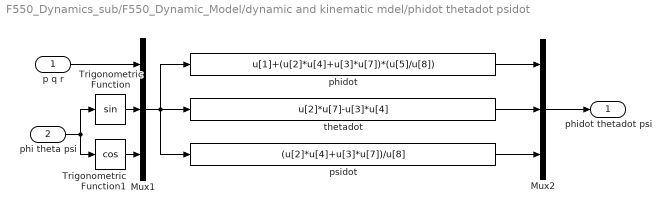
== system F550_Dynamics_sub/F550_Dynamic_Model/dynamic and kinematic mdel/phidot thetadot psidot ==
  p q r : Inport
  phi theta psi : Inport  Port=2
  Mux1 : Mux  Inputs=[3 3 3]
  Mux2 : Mux  Inputs=3
  Trigonometric Function : Trigonometry
  Trigonometric Function1 : Trigonometry  Operator=cos
  phidot : Fcn  Expr=u[1]+(u[2]*u[4]+u[3]*u[7])*(u[5]/u[8])
  psidot : Fcn  Expr=(u[2]*u[4]+u[3]*u[7])/u[8]
  thetadot : Fcn  Expr=u[2]*u[7]-u[3]*u[4]
  phidot thetadot psi : Outport  InitialOutput=0  VectorParamsAs1DForOutWhenUnconnected=off
  wires:
  Trigonometric Function1/1 -> Mux1/3
  Trigonometric Function/1 -> Mux1/2
  Mux2/1 -> phidot thetadot psi/1
  phidot/1 -> Mux2/1
  thetadot/1 -> Mux2/2
  psidot/1 -> Mux2/3
  phi theta psi/1 -> Trigonometric Function1/1, Trigonometric Function/1
  p q r/1 -> Mux1/1
  Mux1/1 -> thetadot/1, phidot/1, psidot/1

== system F550_Dynamics_sub/F550_Dynamic_Model/Ground Model/Crash Detector/norm1 ==
  F : Inport
  Dot Product : DotProduct  OutDataTypeStr=Inherit: Inherit via internal rule
  Sqrt : Sqrt
  Out1 : Outport
  wires:
  Sqrt/1 -> Out1/1
  F/1 -> Dot Product/1, Dot Product/2
  Dot Product/1 -> Sqrt/1

== system F550_Dynamics_sub/F550_Dynamic_Model/Ground Model/Friction Force/Soft Coulomb Friction ==
  note: Pennestrì, E., Rossi, V., Salvini, P. et al. Review and comparison of dry friction force models. Nonlinear Dyn 83, 1785–1801 (2016). https://doi.org/10.1007/s11071-015-2485-3
  In1 : Inport
  Tanh : Trigonometry  Operator=tanh
  friction coefficient : Gain  Gain=contact.translation.friction
  vd : Gain  Gain=1/contact.translation.vd
  Out1 : Outport
  wires:
  friction coefficient/1 -> Out1/1
  Tanh/1 -> friction coefficient/1
  vd/1 -> Tanh/1
  In1/1 -> vd/1

== system F550_Dynamics_sub/F550_Dynamic_Model/Ground Model/Ground Moment Model/Soft Coulomb Friction ==
  note: Pennestrì, E., Rossi, V., Salvini, P. et al. Review and comparison of dry friction force models. Nonlinear Dyn 83, 1785–1801 (2016). https://doi.org/10.1007/s11071-015-2485-3
  In1 : Inport
  Tanh : Trigonometry  Operator=tanh
  friction coefficient : Gain  Gain=control.rotation.friction
  vd : Gain  Gain=1/control.rotation.vd
  Out1 : Outport
  wires:
  friction coefficient/1 -> Out1/1
  Tanh/1 -> friction coefficient/1
  vd/1 -> Tanh/1
  In1/1 -> vd/1

== system F550_Dynamics_sub/F550_Dynamic_Model/Motor Model/MotorNonlinearDynamic1/Motor_Dynamics (1st order) ==
  note: radps_dot = (radps_cmd-radps)/Tm
      | or
      | radps/radps_cmd = 1/(Tm*s +1)
  motor_radps_cmd : Inport
  motor_radps0 : Inport  Port=2
  Add : Sum  Inputs=|+-
  Gain : Gain  Gain=1/motorTm
  Integrator : Integrator  InitialConditionSource=external
  motor_radps : Outport  VectorParamsAs1DForOutWhenUnconnected=off
  wires:
  Add/1 -> Gain/1
  motor_radps0/1 -> Integrator/2
  motor_radps_cmd/1 -> Add/1
  Gain/1 -> Integrator/1  "rads_dot"
  Integrator/1 -> Add/2, motor_radps/1  "radps"

== system F550_Dynamics_sub/F550_Dynamic_Model/Motor Model/MotorNonlinearDynamic2/Motor_Dynamics (1st order) ==
  note: radps_dot = (radps_cmd-radps)/Tm
      | or
      | radps/radps_cmd = 1/(Tm*s +1)
  motor_radps_cmd : Inport
  motor_radps0 : Inport  Port=2
  Add : Sum  Inputs=|+-
  Gain : Gain  Gain=1/motorTm
  Integrator : Integrator  InitialConditionSource=external
  motor_radps : Outport  VectorParamsAs1DForOutWhenUnconnected=off
  wires:
  Integrator/1 -> motor_radps/1, Add/2  "radps"
  Gain/1 -> Integrator/1  "rads_dot"
  motor_radps_cmd/1 -> Add/1
  motor_radps0/1 -> Integrator/2
  Add/1 -> Gain/1

== system F550_Dynamics_sub/F550_Dynamic_Model/Motor Model/MotorNonlinearDynamic3/Motor_Dynamics (1st order) ==
  note: radps_dot = (radps_cmd-radps)/Tm
      | or
      | radps/radps_cmd = 1/(Tm*s +1)
  motor_radps_cmd : Inport
  motor_radps0 : Inport  Port=2
  Add : Sum  Inputs=|+-
  Gain : Gain  Gain=1/motorTm
  Integrator : Integrator  InitialConditionSource=external
  motor_radps : Outport  VectorParamsAs1DForOutWhenUnconnected=off
  wires:
  Add/1 -> Gain/1
  motor_radps0/1 -> Integrator/2
  motor_radps_cmd/1 -> Add/1
  Gain/1 -> Integrator/1  "rads_dot"
  Integrator/1 -> Add/2, motor_radps/1  "radps"

== system F550_Dynamics_sub/F550_Dynamic_Model/Motor Model/MotorNonlinearDynamic4/Motor_Dynamics (1st order) ==
  note: radps_dot = (radps_cmd-radps)/Tm
      | or
      | radps/radps_cmd = 1/(Tm*s +1)
  motor_radps_cmd : Inport
  motor_radps0 : Inport  Port=2
  Add : Sum  Inputs=|+-
  Gain : Gain  Gain=1/motorTm
  Integrator : Integrator  InitialConditionSource=external
  motor_radps : Outport  VectorParamsAs1DForOutWhenUnconnected=off
  wires:
  Integrator/1 -> motor_radps/1, Add/2  "radps"
  Gain/1 -> Integrator/1  "rads_dot"
  motor_radps_cmd/1 -> Add/1
  motor_radps0/1 -> Integrator/2
  Add/1 -> Gain/1

== system F550_Dynamics_sub/F550_Dynamic_Model/Motor Model/MotorNonlinearDynamic5/Motor_Dynamics (1st order) ==
  note: radps_dot = (radps_cmd-radps)/Tm
      | or
      | radps/radps_cmd = 1/(Tm*s +1)
  motor_radps_cmd : Inport
  motor_radps0 : Inport  Port=2
  Add : Sum  Inputs=|+-
  Gain : Gain  Gain=1/motorTm
  Integrator : Integrator  InitialConditionSource=external
  motor_radps : Outport  VectorParamsAs1DForOutWhenUnconnected=off
  wires:
  Integrator/1 -> motor_radps/1, Add/2  "radps"
  Gain/1 -> Integrator/1  "rads_dot"
  motor_radps_cmd/1 -> Add/1
  motor_radps0/1 -> Integrator/2
  Add/1 -> Gain/1

== system F550_Dynamics_sub/F550_Dynamic_Model/Motor Model/MotorNonlinearDynamic6/Motor_Dynamics (1st order) ==
  note: radps_dot = (radps_cmd-radps)/Tm
      | or
      | radps/radps_cmd = 1/(Tm*s +1)
  motor_radps_cmd : Inport
  motor_radps0 : Inport  Port=2
  Add : Sum  Inputs=|+-
  Gain : Gain  Gain=1/motorTm
  Integrator : Integrator  InitialConditionSource=external
  motor_radps : Outport  VectorParamsAs1DForOutWhenUnconnected=off
  wires:
  Integrator/1 -> motor_radps/1, Add/2  "radps"
  Gain/1 -> Integrator/1  "rads_dot"
  motor_radps_cmd/1 -> Add/1
  motor_radps0/1 -> Integrator/2
  Add/1 -> Gain/1

== matlab function F550_Dynamics_sub/F550_Dynamic_Model/Aero Force and Moment ==
  data: Fa output; Ma output; wb input; Vb input; Cd input; Cmd input; dz_cg input
function [Fa,Ma] = fcn(wb,Vb,Cd,Cmd,dz_cg)

 Fa = -Cd*Vb.*abs(Vb);         % Careful for the definition of Cd

 Md = -Cmd.*wb.*abs(wb);       % aerodynamic damping moment
  
 Mfd= [Fa(2)*dz_cg
      -Fa(1)*dz_cg
       0];

 % Ma = Mfd + Md;
 Ma = Md; % Ignore Damping moment
end

== matlab function F550_Dynamics_sub/F550_Dynamic_Model/Euler2DCMbe ==
  data: rpy input; DCMbe output
function DCMbe = fcn(rpy)

phi = rpy(1); theta = rpy(2); psi = rpy(3);
DCMbe = [ cos(psi)*cos(theta), sin(psi)*cos(theta), -sin(theta);
      -sin(psi)*cos(phi)+cos(psi)*sin(theta)*sin(phi), cos(psi)*cos(phi)+sin(psi)*sin(theta)*sin(phi), cos(theta)*sin(phi);
      sin(psi)*sin(phi)+cos(psi)*sin(theta)*cos(phi), -cos(psi)*sin(phi)+sin(psi)*sin(theta)*cos(phi), cos(theta)*cos(phi);
];

== matlab function F550_Dynamics_sub/F550_Dynamic_Model/F450 Quadcopter Prop Force and Moment1 ==
  data: w input; R input; Cm input; Ct input; Fprop output; Mprop output; wb input; Jrp input
function [Fprop, Mprop] = fcn(w, R, Cm, Ct, wb, Jrp)

 %  Obtain the force and torque acting on the body. 
 %  The airframe of the quadrotor is as follows:
 %  3↓   1↑
 %    \ /
 %    / \
 %  2↑   4↓
 %  ↑ stands for counterclockwise and ↓stands for clockwise.
 
 % Input：
 %  w: motor speed，unit：rad/s
 %  R: body radius(m)
 %  Cm: torque coefficient
 %  Ct: thrust coefficient
 %  wb: angular velocity in the body coordinate system
 %  Jrp:  moment of inertia of motor rotor + propeller

 % Output:
 %  Fprop: force vector from prop
 %  Mprop: aerodynamic damping moment + gyro moment

 
 F_prop = Ct*(w.^2);      % Force from each prop
 M_prop = Cm*(w.^2);      % Torque magnitude from each prop

 Fprop = [0; 0; -sum(F_prop)];

 d=sin(pi/4)*R;
 Mp= [ d*F_prop'*[-1;  1;  1; -1]
       d*F_prop'*[ 1; -1;  1; -1]
         M_prop'*[ 1;  1; -1; -1] ];

% gyro moment
 M_gyro   = [Jrp*wb(2)*( w(1) + w(2) - w(3) - w(4));  
             Jrp*wb(1)*(-w(1) - w(2) + w(3) + w(4));
             0];

 Mprop = Mp + M_gyro;

end

== matlab function F550_Dynamics_sub/F550_Dynamic_Model/F550 Hexacopter Prop Force and Moment ==
  data: w input; L input; Cm input; Ct input; Fprop output; Mprop output; wb input; Jrp input
function [Fprop, Mprop] = fcn(w, L, Cm, Ct, wb, Jrp)

 % Body Frame : NED Coordinate
 % X-axis : Heading, Y-axis : Right wing, Z-axis : Down

 %  Obtain the force and torque acting on the body. 
 %  The airframe of the hexarotor is as follows: PX4 Hexacopter Configuration
 %     3↓   5↑
 %      \  /
 %   2↑--  -- 1↓
 %      /  \
 %     6↓   4↑
 %  ↑ stands for counterclockwise and ↓stands for clockwise.


 % Input：
 %  w: motor speed，unit：rad/s
 %  L: Arm Length (m) - In case of F550 R = 0.275 m
 %  Cm: torque coefficient
 %  Ct: thrust coefficient
 %  wb: angular velocity in the body coordinate system
 %  Jrp:  moment of inertia of motor rotor + propeller

 % Output:
 %  Fprop: force vector from prop
 %  Mprop: aerodynamic damping moment + gyro moment
        
        % Legacy Code - From F450 Quadcopter 
        %  F_prop = Ct*(w.^2);      % Force from each prop
        %  M_prop = Cm*(w.^2);      % Torque magnitude from each prop
        % 
        %  Fprop = [0; 0; -sum(F_prop)];
        % 
        %  d=sin(pi/4)*R;
        %  Mp= [ d*F_prop'*[-1;  1;  1; -1]
        %        d*F_prop'*[ 1; -1;  1; -1]
        %          M_prop'*[ 1;  1; -1; -1] ];
        % 
        % % gyro moment
        %  M_gyro   = [Jrp*wb(2)*( w(1) + w(2) - w(3) - w(4));  
        %              Jrp*wb(1)*(-w(1) - w(2) + w(3) + w(4));
        %              0];
        % 
        %  Mprop = Mp + M_gyro;
    
    % 로터 회전수에 따른 추력 및 모멘트
    F_prop = Ct * (w.^2);
    M_prop = Cm * (w.^2);
    
    % 프로펠러에 의한 힘 
    Fprop = [0; 0; -sum(F_prop)];
    
    % 로터에 추력/회전에 의해 기체에 작용하는 모멘트
    Mp = [ F_prop'*[-L; L; 0.5*L; -0.5*L; -0.5*L; 0.5*L]
           F_prop'*[0; 0; sqrt(3)/2*L; -sqrt(3)/2*L; sqrt(3)/2*L; -sqrt(3)/2*L]
           M_prop'*[-1; 1; -1; 1; -1; 1;]
         ];
    
    % 동체 회전에 의해 회전하는 프롭에 작용하는 모멘트
    M_gyro = [Jrp*wb(2)*( -w(1)+w(2)-w(3)+w(4)-w(5)+w(6) );
              -Jrp*wb(1)*( -w(1)+w(2)-w(3)+w(4)-w(5)+w(6));
              0;
        ];
    
    Mprop = Mp + M_gyro;
end
